simulink model "fft32kpt_ssr32_float"  (R2024a)
settings: Solver=VariableStepAuto  StartTime=0.0  StopTime=sample_period*N*6  RelTol=1e-3
PreLoadFcn:
  | clk_freq = 570e6;
  | SSR=32; % transpose block SSR settings...
  | sample_period = 1/(SSR*clk_freq);
  | N=32768; % fft point size
  | binw=(1/sample_period) / (2*N); % bin width
  | bin_freq = 2*pi*3*binw+pi*binw; % sin, cos freq centered in channel
  | 
  | % for transpose block
  | DATA_WIDTH=32;
  | M=32;
  | N1=N/M;
  | MEM_STYLE=4; % MEM OPTIONS: 4 - ULTRA, 0 - AUTO, 1 - BRAM, 5 - MIXED
InitFcn:
  | clk_freq = 570e6;
  | SSR=32; % transpose block SSR settings...
  | sample_period = 1/(SSR*clk_freq);
  | N=32768; % fft point size
  | binw=(1/sample_period) / (2*N); % bin width
  | bin_freq = 2*pi*3*binw+pi*binw; % sin, cos freq centered in channel
  | 
  | % for transpose block
  | DATA_WIDTH=32;
  | M=32;
  | N1=N/M;
  | MEM_STYLE=4; % MEM OPTIONS: 4 - ULTRA, 0 - AUTO, 1 - BRAM, 5 - MIXED
undefined symbols (not defined in the file or in its folder): None, S, vsva2197, xcvc1902
libraries: hdlBasic x139, aieBasic x95, aieUtilities x32, aieDSP x32, hdlUtilities x32, matrix_library x32, hdlSSR x12, hdlDSPIP x1, simulink x1, dspxfrm3 x1, vmcUtilities x1
(part 4 of 4)

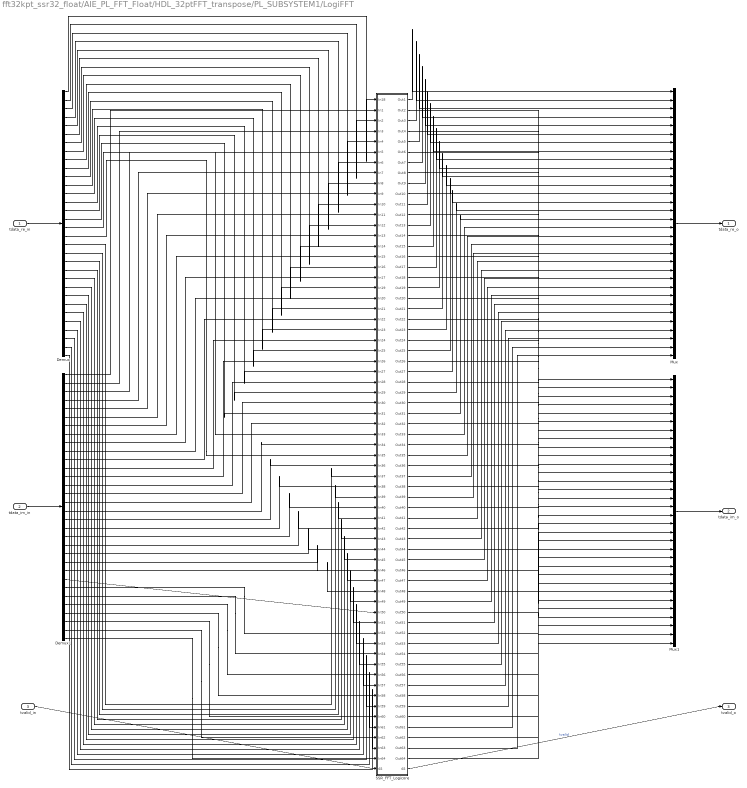
== system fft32kpt_ssr32_float/AIE_PL_FFT_Float/HDL_32ptFFT_transpose/PL_SUBSYSTEM1/LogiFFT ==
  tdata_re_in : Inport
  tdata_im_in : Inport  Port=2
  tvalid_in : Inport  Port=3
  Demux : Demux  Outputs=32
  Demux1 : Demux  Outputs=32
  Mux : Mux  Inputs=32
  Mux1 : Mux  Inputs=32
  SSR_FFT_Logicore : Subsystem
  tdata_re_o : Outport
  tdata_im_o : Outport  Port=2
  tvalid_o : Outport  Port=3
  wires:
  SSR_FFT_Logicore/2(Out2) -> Mux1/1
  SSR_FFT_Logicore/4(Out4) -> Mux1/2
  SSR_FFT_Logicore/6(Out6) -> Mux1/3
  SSR_FFT_Logicore/8(Out8) -> Mux1/4
  SSR_FFT_Logicore/10(Out10) -> Mux1/5
  SSR_FFT_Logicore/12(Out12) -> Mux1/6
  SSR_FFT_Logicore/14(Out14) -> Mux1/7
  SSR_FFT_Logicore/16(Out16) -> Mux1/8
  SSR_FFT_Logicore/18(Out18) -> Mux1/9
  SSR_FFT_Logicore/20(Out20) -> Mux1/10
  SSR_FFT_Logicore/22(Out22) -> Mux1/11
  SSR_FFT_Logicore/24(Out24) -> Mux1/12
  SSR_FFT_Logicore/26(Out26) -> Mux1/13
  SSR_FFT_Logicore/28(Out28) -> Mux1/14
  SSR_FFT_Logicore/30(Out30) -> Mux1/15
  SSR_FFT_Logicore/32(Out32) -> Mux1/16
  SSR_FFT_Logicore/34(Out34) -> Mux1/17
  SSR_FFT_Logicore/36(Out36) -> Mux1/18
  SSR_FFT_Logicore/38(Out38) -> Mux1/19
  SSR_FFT_Logicore/64(Out64) -> Mux1/32
  SSR_FFT_Logicore/40(Out40) -> Mux1/20
  SSR_FFT_Logicore/62(Out62) -> Mux1/31
  SSR_FFT_Logicore/42(Out42) -> Mux1/21
  SSR_FFT_Logicore/60(Out60) -> Mux1/30
  SSR_FFT_Logicore/44(Out44) -> Mux1/22
  SSR_FFT_Logicore/58(Out58) -> Mux1/29
  SSR_FFT_Logicore/46(Out46) -> Mux1/23
  SSR_FFT_Logicore/56(Out56) -> Mux1/28
  SSR_FFT_Logicore/48(Out48) -> Mux1/24
  SSR_FFT_Logicore/54(Out54) -> Mux1/27
  SSR_FFT_Logicore/50(Out50) -> Mux1/25
  SSR_FFT_Logicore/52(Out52) -> Mux1/26
  SSR_FFT_Logicore/63(Out63) -> Mux/32
  SSR_FFT_Logicore/61(Out61) -> Mux/31
  SSR_FFT_Logicore/59(Out59) -> Mux/30
  SSR_FFT_Logicore/57(Out57) -> Mux/29
  SSR_FFT_Logicore/55(Out55) -> Mux/28
  SSR_FFT_Logicore/53(Out53) -> Mux/27
  SSR_FFT_Logicore/51(Out51) -> Mux/26
  SSR_FFT_Logicore/49(Out49) -> Mux/25
  SSR_FFT_Logicore/47(Out47) -> Mux/24
  SSR_FFT_Logicore/45(Out45) -> Mux/23
  SSR_FFT_Logicore/43(Out43) -> Mux/22
  SSR_FFT_Logicore/41(Out41) -> Mux/21
  SSR_FFT_Logicore/39(Out39) -> Mux/20
  SSR_FFT_Logicore/37(Out37) -> Mux/19
  SSR_FFT_Logicore/35(Out35) -> Mux/18
  SSR_FFT_Logicore/33(Out33) -> Mux/17
  SSR_FFT_Logicore/31(Out31) -> Mux/16
  SSR_FFT_Logicore/29(Out29) -> Mux/15
  SSR_FFT_Logicore/27(Out27) -> Mux/14
  SSR_FFT_Logicore/25(Out25) -> Mux/13
  SSR_FFT_Logicore/23(Out23) -> Mux/12
  SSR_FFT_Logicore/21(Out21) -> Mux/11
  SSR_FFT_Logicore/19(Out19) -> Mux/10
  SSR_FFT_Logicore/17(Out17) -> Mux/9
  SSR_FFT_Logicore/15(Out15) -> Mux/8
  SSR_FFT_Logicore/13(Out13) -> Mux/7
  SSR_FFT_Logicore/11(Out11) -> Mux/6
  SSR_FFT_Logicore/9(Out9) -> Mux/5
  SSR_FFT_Logicore/7(Out7) -> Mux/4
  SSR_FFT_Logicore/5(Out5) -> Mux/3
  SSR_FFT_Logicore/3(Out3) -> Mux/2
  SSR_FFT_Logicore/1(Out1) -> Mux/1
  Mux1/1 -> tdata_im_o/1
  Demux1/1 -> SSR_FFT_Logicore/2(In1)
  Demux1/2 -> SSR_FFT_Logicore/4(In3)
  Demux1/3 -> SSR_FFT_Logicore/6(In5)
  Demux1/4 -> SSR_FFT_Logicore/8(In7)
  Demux1/5 -> SSR_FFT_Logicore/10(In9)
  Demux1/6 -> SSR_FFT_Logicore/12(In11)
  Demux1/7 -> SSR_FFT_Logicore/14(In13)
  Demux1/8 -> SSR_FFT_Logicore/16(In15)
  Demux1/9 -> SSR_FFT_Logicore/18(In17)
  Demux1/10 -> SSR_FFT_Logicore/20(In20)
  Demux1/11 -> SSR_FFT_Logicore/22(In22)
  Demux1/12 -> SSR_FFT_Logicore/24(In24)
  Demux1/13 -> SSR_FFT_Logicore/26(In26)
  Demux1/14 -> SSR_FFT_Logicore/28(In28)
  Demux1/15 -> SSR_FFT_Logicore/30(In30)
  Demux1/16 -> SSR_FFT_Logicore/32(In32)
  Demux1/17 -> SSR_FFT_Logicore/34(In34)
  Demux1/32 -> SSR_FFT_Logicore/64(In64)
  Demux1/18 -> SSR_FFT_Logicore/36(In36)
  Demux1/31 -> SSR_FFT_Logicore/62(In62)
  Demux1/19 -> SSR_FFT_Logicore/38(In38)
  Demux1/30 -> SSR_FFT_Logicore/60(In60)
  Demux1/20 -> SSR_FFT_Logicore/40(In40)
  Demux1/29 -> SSR_FFT_Logicore/58(In58)
  Demux1/21 -> SSR_FFT_Logicore/42(In42)
  Demux1/28 -> SSR_FFT_Logicore/56(In56)
  Demux1/22 -> SSR_FFT_Logicore/44(In44)
  Demux1/27 -> SSR_FFT_Logicore/54(In54)
  Demux1/23 -> SSR_FFT_Logicore/46(In46)
  Demux1/26 -> SSR_FFT_Logicore/52(In52)
  Demux1/24 -> SSR_FFT_Logicore/48(In48)
  Demux1/25 -> SSR_FFT_Logicore/50(In50)
  Demux/32 -> SSR_FFT_Logicore/63(In63)
  Demux/31 -> SSR_FFT_Logicore/61(In61)
  Demux/30 -> SSR_FFT_Logicore/59(In59)
  Demux/29 -> SSR_FFT_Logicore/57(In57)
  Demux/28 -> SSR_FFT_Logicore/55(In55)
  Demux/27 -> SSR_FFT_Logicore/53(In53)
  Demux/26 -> SSR_FFT_Logicore/51(In51)
  Demux/25 -> SSR_FFT_Logicore/49(In49)
  Demux/24 -> SSR_FFT_Logicore/47(In47)
  Demux/23 -> SSR_FFT_Logicore/45(In45)
  Demux/22 -> SSR_FFT_Logicore/43(In43)
  Demux/21 -> SSR_FFT_Logicore/41(In41)
  Demux/20 -> SSR_FFT_Logicore/39(In39)
  Demux/19 -> SSR_FFT_Logicore/37(In37)
  Demux/18 -> SSR_FFT_Logicore/35(In35)
  Demux/17 -> SSR_FFT_Logicore/33(In33)
  Demux/16 -> SSR_FFT_Logicore/31(In31)
  Demux/15 -> SSR_FFT_Logicore/29(In29)
  Demux/14 -> SSR_FFT_Logicore/27(In27)
  Demux/13 -> SSR_FFT_Logicore/25(In25)
  Demux/12 -> SSR_FFT_Logicore/23(In23)
  Demux/11 -> SSR_FFT_Logicore/21(In21)
  Demux/10 -> SSR_FFT_Logicore/19(In19)
  Demux/9 -> SSR_FFT_Logicore/17(In16)
  Demux/8 -> SSR_FFT_Logicore/15(In14)
  Demux/7 -> SSR_FFT_Logicore/13(In12)
  Demux/6 -> SSR_FFT_Logicore/11(In10)
  Demux/5 -> SSR_FFT_Logicore/9(In8)
  Demux/4 -> SSR_FFT_Logicore/7(In6)
  Demux/3 -> SSR_FFT_Logicore/5(In4)
  Demux/2 -> SSR_FFT_Logicore/3(In2)
  Demux/1 -> SSR_FFT_Logicore/1(In18)
  tdata_im_in/1 -> Demux1/1
  tvalid_in/1 -> SSR_FFT_Logicore/65(tvalid_in)
  tdata_re_in/1 -> Demux/1
  SSR_FFT_Logicore/65(tvalid_o) -> tvalid_o/1  "tvalid"
  Mux/1 -> tdata_re_o/1

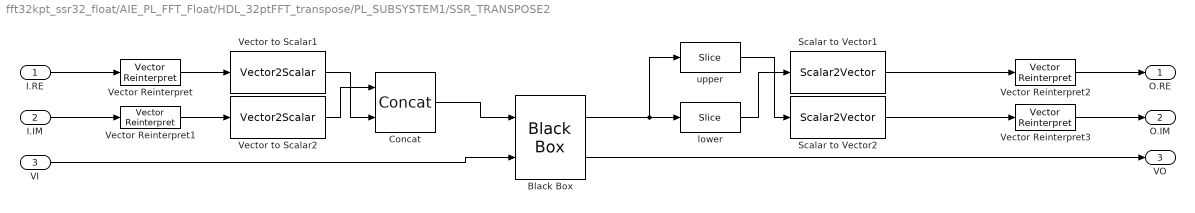
== system fft32kpt_ssr32_float/AIE_PL_FFT_Float/HDL_32ptFFT_transpose/PL_SUBSYSTEM1/SSR_TRANSPOSE2 ==
  "I.RE " : Inport
  "I.IM " : Inport  Port=2
  "VI " : Inport  Port=3
  Black Box : hdlBasic/Black Box  init_code=ssr_transpose_top_config  sim_method=Vivado Simulator  engine_block=../../Questa  verbose=on  XmcBlockStatus=1  maskContainerNames=group1  block_type=blackbox2  block_config=sysgen:black_box_config
  Concat : hdlBasic/Concat  num_inputs=2  XmcBlockStatus=1  maskContainerNames=group1  block_type=concat  block_config=sysgen:Concat_config
  Scalar to Vector1 : hdlSSR/Scalar2Vector  Width=DATA_WIDTH  sg_ssr=SSR  block_type=scalar2vector_ssr  XmcBlockStatus=1  sg_ssr_prev=32  maskContainerNames=group1
  Scalar to Vector2 : hdlSSR/Scalar2Vector  Width=DATA_WIDTH  sg_ssr=SSR  block_type=scalar2vector_ssr  XmcBlockStatus=1  sg_ssr_prev=32  maskContainerNames=group1
  Vector Reinterpret : hdlSSR/Vector Reinterpret  force_arith_type=on  arith_type=Unsigned  force_bin_pt=on  bin_pt=0  sg_ssr=SSR  block_type=reinterpret_ssr  XmcBlockStatus=1  sg_ssr_prev=32  maskContainerNames=group1
  Vector Reinterpret1 : hdlSSR/Vector Reinterpret  force_arith_type=on  arith_type=Unsigned  force_bin_pt=on  bin_pt=0  sg_ssr=SSR  block_type=reinterpret_ssr  XmcBlockStatus=1  sg_ssr_prev=32  maskContainerNames=group1
  Vector Reinterpret2 : hdlSSR/Vector Reinterpret  force_arith_type=on  arith_type=Floating-point  force_bin_pt=on  bin_pt=24  sg_ssr=SSR  block_type=reinterpret_ssr  XmcBlockStatus=1  sg_ssr_prev=32  maskContainerNames=group1
  Vector Reinterpret3 : hdlSSR/Vector Reinterpret  force_arith_type=on  arith_type=Floating-point  force_bin_pt=on  bin_pt=24  sg_ssr=SSR  block_type=reinterpret_ssr  XmcBlockStatus=1  sg_ssr_prev=32  maskContainerNames=group1
  Vector to Scalar1 : hdlSSR/Vector2Scalar  sg_ssr=SSR  block_type=vector2scalar_ssr  XmcBlockStatus=1  sg_ssr_prev=32  maskContainerNames=group1
  Vector to Scalar2 : hdlSSR/Vector2Scalar  sg_ssr=SSR  block_type=vector2scalar_ssr  XmcBlockStatus=1  sg_ssr_prev=32  maskContainerNames=group1
  lower : hdlBasic/Slice  nbits=DATA_WIDTH*SSR  boolean_output=off  mode=Lower Bit Location + Width  bit1=0  base1=MSB of Input  bit0=0  base0=LSB of Input  XmcBlockStatus=1  maskContainerNames=group1  block_type=slice  block_config=sysgen:Slice_config
  upper : hdlBasic/Slice  nbits=DATA_WIDTH*SSR  boolean_output=off  mode=Upper Bit Location + Width  bit1=0  base1=MSB of Input  bit0=0  base0=LSB of Input  XmcBlockStatus=1  maskContainerNames=group1  block_type=slice  block_config=sysgen:Slice_config
  " O.RE" : Outport
  " O.IM" : Outport  Port=2
  " VO" : Outport  Port=3
  wires:
  Vector Reinterpret3/1 -> " O.IM"/1
  Vector Reinterpret2/1 -> " O.RE"/1
  Vector Reinterpret/1 -> Vector to Scalar1/1
  "VI "/1 -> Black Box/2
  Vector to Scalar1/1 -> Concat/2
  lower/1 -> Scalar to Vector1/1
  upper/1 -> Scalar to Vector2/1
  Black Box/1 -> lower/1, upper/1
  Vector to Scalar2/1 -> Concat/1
  Concat/1 -> Black Box/1
  Vector Reinterpret1/1 -> Vector to Scalar2/1
  Black Box/2 -> " VO"/1
  Scalar to Vector1/1 -> Vector Reinterpret2/1
  Scalar to Vector2/1 -> Vector Reinterpret3/1
  "I.RE "/1 -> Vector Reinterpret/1
  "I.IM "/1 -> Vector Reinterpret1/1

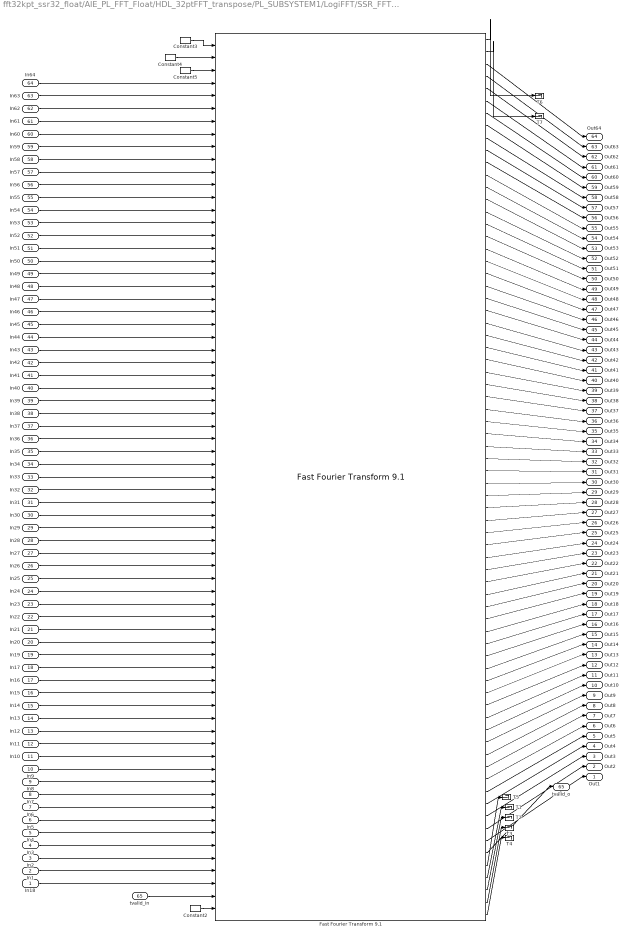
== system fft32kpt_ssr32_float/AIE_PL_FFT_Float/HDL_32ptFFT_transpose/PL_SUBSYSTEM1/LogiFFT/SSR_FFT_Logicore ==
  In18 : Inport
  In1 : Inport  Port=2
  In2 : Inport  Port=3
  In3 : Inport  Port=4
  In4 : Inport  Port=5
  In5 : Inport  Port=6
  In6 : Inport  Port=7
  In7 : Inport  Port=8
  In8 : Inport  Port=9
  In9 : Inport  Port=10
  In10 : Inport  Port=11
  In11 : Inport  Port=12
  In12 : Inport  Port=13
  In13 : Inport  Port=14
  In14 : Inport  Port=15
  In15 : Inport  Port=16
  In16 : Inport  Port=17
  In17 : Inport  Port=18
  In19 : Inport  Port=19
  In20 : Inport  Port=20
  In21 : Inport  Port=21
  In22 : Inport  Port=22
  In23 : Inport  Port=23
  In24 : Inport  Port=24
  In25 : Inport  Port=25
  In26 : Inport  Port=26
  In27 : Inport  Port=27
  In28 : Inport  Port=28
  In29 : Inport  Port=29
  In30 : Inport  Port=30
  In31 : Inport  Port=31
  In32 : Inport  Port=32
  In33 : Inport  Port=33
  In34 : Inport  Port=34
  In35 : Inport  Port=35
  In36 : Inport  Port=36
  In37 : Inport  Port=37
  In38 : Inport  Port=38
  In39 : Inport  Port=39
  In40 : Inport  Port=40
  In41 : Inport  Port=41
  In42 : Inport  Port=42
  In43 : Inport  Port=43
  In44 : Inport  Port=44
  In45 : Inport  Port=45
  In46 : Inport  Port=46
  In47 : Inport  Port=47
  In48 : Inport  Port=48
  In49 : Inport  Port=49
  In50 : Inport  Port=50
  In51 : Inport  Port=51
  In52 : Inport  Port=52
  In53 : Inport  Port=53
  In54 : Inport  Port=54
  In55 : Inport  Port=55
  In56 : Inport  Port=56
  In57 : Inport  Port=57
  In58 : Inport  Port=58
  In59 : Inport  Port=59
  In60 : Inport  Port=60
  In61 : Inport  Port=61
  In62 : Inport  Port=62
  In63 : Inport  Port=63
  In64 : Inport  Port=64
  tvalid_in : Inport  Port=65
  Constant2 : hdlBasic/Constant  const=0  gui_display_data_type=Boolean  arith_type=Boolean  n_bits=16  bin_pt=14  preci_type=Single  exp_width=8  frac_width=24  explicit_period=off  period=1  XmcBlockStatus=1  maskContainerNames=tabcontainer1  block_type=constant  block_config=sysgen:Constant_config
  Constant3 : hdlBasic/Constant  const=0  gui_display_data_type=Fixed-point  arith_type=Unsigned  n_bits=6  bin_pt=0  preci_type=Single  exp_width=8  frac_width=24  explicit_period=off  period=1  XmcBlockStatus=1  maskContainerNames=tabcontainer1  block_type=constant  block_config=sysgen:Constant_config
  Constant4 : hdlBasic/Constant  const=1.0  gui_display_data_type=Fixed-point  arith_type=Unsigned  n_bits=1  bin_pt=0  preci_type=Single  exp_width=8  frac_width=24  explicit_period=off  period=1  XmcBlockStatus=1  maskContainerNames=tabcontainer1  block_type=constant  block_config=sysgen:Constant_config
  Constant5 : hdlBasic/Constant  const=0  gui_display_data_type=Boolean  arith_type=Boolean  n_bits=16  bin_pt=14  preci_type=Single  exp_width=8  frac_width=24  explicit_period=off  period=1  XmcBlockStatus=1  maskContainerNames=tabcontainer1  block_type=constant  block_config=sysgen:Constant_config
  Fast Fourier Transform 9.1 : hdlDSPIP/Fast Fourier Transform 9.1   transform_length=32  target_clock_frequency=clk_freq/1e6  target_data_throughput=clk_freq/1e6  implementation_options=automatically_select  run_time_configurable_transform_length=off  enable_ssr=on  super_sample_rates=32  data_format=native_floating_point  phase_factor_width=18  scaling_options=scaled  rounding_modes=truncation  aclken=off  aresetn=off  output_ordering=bit_reversed_order  cyclic_prefix_insertion=off  throttle_scheme=realtime  xk_index=off  ovflo=off  trim_axipin_name=on  memory_options_data=block_ram  memory_options_phase_factors=block_ram  number_of_stages_using_block_ram_for_data_and_phase_factors=0  memory_options_reorder=block_ram  memory_options_hybrid=off  complex_mult_type=use_mults_resources  butterfly_type=use_luts  simulation_type=hybrid  simulation_model=sysgen:xfftv9_cmodel  data_path_portlist={ 's_axis_data_tdata', 'm_axis_data_tdata', 'm_axis_status_tdata', 'event_fft_overflow' }  channels=1  input_ordering=natural_order  input_width=16  ip_name=Fast Fourier Transform  ip_version=9.1  dsptool_ready=true  ipcore_usecache=true  ipcore_useipmodelcache=true  wrapper_available=true  port_translation_map={ 'aclken' => 'en', 'aresetn' => 'rst'}  XmcBlockStatus=1  maskContainerNames=tabcontainer1  block_type=xfft_v9_1  block_config=sysgen:rodinimport_config
  T{1..7} (7 alike) : Terminator
  Out1 : Outport
  Out2 : Outport  Port=2
  Out3 : Outport  Port=3
  Out4 : Outport  Port=4
  Out5 : Outport  Port=5
  Out6 : Outport  Port=6
  Out7 : Outport  Port=7
  Out8 : Outport  Port=8
  Out9 : Outport  Port=9
  Out10 : Outport  Port=10
  Out11 : Outport  Port=11
  Out12 : Outport  Port=12
  Out13 : Outport  Port=13
  Out14 : Outport  Port=14
  Out15 : Outport  Port=15
  Out16 : Outport  Port=16
  Out17 : Outport  Port=17
  Out18 : Outport  Port=18
  Out19 : Outport  Port=19
  Out20 : Outport  Port=20
  Out21 : Outport  Port=21
  Out22 : Outport  Port=22
  Out23 : Outport  Port=23
  Out24 : Outport  Port=24
  Out25 : Outport  Port=25
  Out26 : Outport  Port=26
  Out27 : Outport  Port=27
  Out28 : Outport  Port=28
  Out29 : Outport  Port=29
  Out30 : Outport  Port=30
  Out31 : Outport  Port=31
  Out32 : Outport  Port=32
  Out33 : Outport  Port=33
  Out34 : Outport  Port=34
  Out35 : Outport  Port=35
  Out36 : Outport  Port=36
  Out37 : Outport  Port=37
  Out38 : Outport  Port=38
  Out39 : Outport  Port=39
  Out40 : Outport  Port=40
  Out41 : Outport  Port=41
  Out42 : Outport  Port=42
  Out43 : Outport  Port=43
  Out44 : Outport  Port=44
  Out45 : Outport  Port=45
  Out46 : Outport  Port=46
  Out47 : Outport  Port=47
  Out48 : Outport  Port=48
  Out49 : Outport  Port=49
  Out50 : Outport  Port=50
  Out51 : Outport  Port=51
  Out52 : Outport  Port=52
  Out53 : Outport  Port=53
  Out54 : Outport  Port=54
  Out55 : Outport  Port=55
  Out56 : Outport  Port=56
  Out57 : Outport  Port=57
  Out58 : Outport  Port=58
  Out59 : Outport  Port=59
  Out60 : Outport  Port=60
  Out61 : Outport  Port=61
  Out62 : Outport  Port=62
  Out63 : Outport  Port=63
  Out64 : Outport  Port=64
  tvalid_o : Outport  Port=65
  wires:
  Fast Fourier Transform 9.1/66 -> Out1/1
  Fast Fourier Transform 9.1/65 -> Out2/1
  Fast Fourier Transform 9.1/64 -> Out3/1
  Fast Fourier Transform 9.1/63 -> Out4/1
  Fast Fourier Transform 9.1/62 -> Out5/1
  Fast Fourier Transform 9.1/61 -> Out6/1
  Fast Fourier Transform 9.1/60 -> Out7/1
  Fast Fourier Transform 9.1/59 -> Out8/1
  Fast Fourier Transform 9.1/58 -> Out9/1
  Fast Fourier Transform 9.1/57 -> Out10/1
  Fast Fourier Transform 9.1/56 -> Out11/1
  Fast Fourier Transform 9.1/55 -> Out12/1
  Fast Fourier Transform 9.1/54 -> Out13/1
  Fast Fourier Transform 9.1/53 -> Out14/1
  Fast Fourier Transform 9.1/52 -> Out15/1
  Fast Fourier Transform 9.1/51 -> Out16/1
  Fast Fourier Transform 9.1/50 -> Out17/1
  Fast Fourier Transform 9.1/49 -> Out18/1
  Fast Fourier Transform 9.1/48 -> Out19/1
  Fast Fourier Transform 9.1/47 -> Out20/1
  Fast Fourier Transform 9.1/46 -> Out21/1
  Fast Fourier Transform 9.1/45 -> Out22/1
  Fast Fourier Transform 9.1/44 -> Out23/1
  Fast Fourier Transform 9.1/43 -> Out24/1
  Fast Fourier Transform 9.1/42 -> Out25/1
  Fast Fourier Transform 9.1/41 -> Out26/1
  Fast Fourier Transform 9.1/40 -> Out27/1
  Fast Fourier Transform 9.1/39 -> Out28/1
  Fast Fourier Transform 9.1/38 -> Out29/1
  Fast Fourier Transform 9.1/37 -> Out30/1
  Fast Fourier Transform 9.1/36 -> Out31/1
  Fast Fourier Transform 9.1/35 -> Out32/1
  Fast Fourier Transform 9.1/34 -> Out33/1
  Fast Fourier Transform 9.1/33 -> Out34/1
  Fast Fourier Transform 9.1/32 -> Out35/1
  Fast Fourier Transform 9.1/31 -> Out36/1
  Fast Fourier Transform 9.1/30 -> Out37/1
  Fast Fourier Transform 9.1/29 -> Out38/1
  Fast Fourier Transform 9.1/28 -> Out39/1
  Fast Fourier Transform 9.1/27 -> Out40/1
  Fast Fourier Transform 9.1/26 -> Out41/1
  Fast Fourier Transform 9.1/25 -> Out42/1
  Fast Fourier Transform 9.1/24 -> Out43/1
  Fast Fourier Transform 9.1/23 -> Out44/1
  Fast Fourier Transform 9.1/22 -> Out45/1
  Fast Fourier Transform 9.1/21 -> Out46/1
  Fast Fourier Transform 9.1/20 -> Out47/1
  Fast Fourier Transform 9.1/19 -> Out48/1
  Fast Fourier Transform 9.1/18 -> Out49/1
  Fast Fourier Transform 9.1/17 -> Out50/1
  Fast Fourier Transform 9.1/16 -> Out51/1
  Fast Fourier Transform 9.1/15 -> Out52/1
  Fast Fourier Transform 9.1/14 -> Out53/1
  Fast Fourier Transform 9.1/13 -> Out54/1
  Fast Fourier Transform 9.1/12 -> Out55/1
  Fast Fourier Transform 9.1/11 -> Out56/1
  Fast Fourier Transform 9.1/10 -> Out57/1
  Fast Fourier Transform 9.1/9 -> Out58/1
  Fast Fourier Transform 9.1/8 -> Out59/1
  Fast Fourier Transform 9.1/7 -> Out60/1
  Fast Fourier Transform 9.1/6 -> Out61/1
  Fast Fourier Transform 9.1/5 -> Out62/1
  Fast Fourier Transform 9.1/4 -> Out63/1
  Fast Fourier Transform 9.1/3 -> Out64/1
  tvalid_in/1 -> Fast Fourier Transform 9.1/68
  In18/1 -> Fast Fourier Transform 9.1/67
  In1/1 -> Fast Fourier Transform 9.1/66
  In2/1 -> Fast Fourier Transform 9.1/65
  In3/1 -> Fast Fourier Transform 9.1/64
  In4/1 -> Fast Fourier Transform 9.1/63
  In5/1 -> Fast Fourier Transform 9.1/62
  In6/1 -> Fast Fourier Transform 9.1/61
  In7/1 -> Fast Fourier Transform 9.1/60
  In8/1 -> Fast Fourier Transform 9.1/59
  In9/1 -> Fast Fourier Transform 9.1/58
  In10/1 -> Fast Fourier Transform 9.1/57
  In11/1 -> Fast Fourier Transform 9.1/56
  In12/1 -> Fast Fourier Transform 9.1/55
  In13/1 -> Fast Fourier Transform 9.1/54
  In14/1 -> Fast Fourier Transform 9.1/53
  In15/1 -> Fast Fourier Transform 9.1/52
  In16/1 -> Fast Fourier Transform 9.1/51
  In17/1 -> Fast Fourier Transform 9.1/50
  In19/1 -> Fast Fourier Transform 9.1/49
  In20/1 -> Fast Fourier Transform 9.1/48
  In21/1 -> Fast Fourier Transform 9.1/47
  In22/1 -> Fast Fourier Transform 9.1/46
  In23/1 -> Fast Fourier Transform 9.1/45
  In24/1 -> Fast Fourier Transform 9.1/44
  In25/1 -> Fast Fourier Transform 9.1/43
  In26/1 -> Fast Fourier Transform 9.1/42
  In27/1 -> Fast Fourier Transform 9.1/41
  In28/1 -> Fast Fourier Transform 9.1/40
  In29/1 -> Fast Fourier Transform 9.1/39
  In30/1 -> Fast Fourier Transform 9.1/38
  In31/1 -> Fast Fourier Transform 9.1/37
  In32/1 -> Fast Fourier Transform 9.1/36
  In33/1 -> Fast Fourier Transform 9.1/35
  In34/1 -> Fast Fourier Transform 9.1/34
  In35/1 -> Fast Fourier Transform 9.1/33
  In36/1 -> Fast Fourier Transform 9.1/32
  In37/1 -> Fast Fourier Transform 9.1/31
  In38/1 -> Fast Fourier Transform 9.1/30
  In39/1 -> Fast Fourier Transform 9.1/29
  In40/1 -> Fast Fourier Transform 9.1/28
  In41/1 -> Fast Fourier Transform 9.1/27
  In42/1 -> Fast Fourier Transform 9.1/26
  In43/1 -> Fast Fourier Transform 9.1/25
  In44/1 -> Fast Fourier Transform 9.1/24
  In45/1 -> Fast Fourier Transform 9.1/23
  In46/1 -> Fast Fourier Transform 9.1/22
  In47/1 -> Fast Fourier Transform 9.1/21
  In48/1 -> Fast Fourier Transform 9.1/20
  In49/1 -> Fast Fourier Transform 9.1/19
  In50/1 -> Fast Fourier Transform 9.1/18
  In51/1 -> Fast Fourier Transform 9.1/17
  In52/1 -> Fast Fourier Transform 9.1/16
  In53/1 -> Fast Fourier Transform 9.1/15
  In54/1 -> Fast Fourier Transform 9.1/14
  In55/1 -> Fast Fourier Transform 9.1/13
  In56/1 -> Fast Fourier Transform 9.1/12
  In57/1 -> Fast Fourier Transform 9.1/11
  In58/1 -> Fast Fourier Transform 9.1/10
  In59/1 -> Fast Fourier Transform 9.1/9
  In60/1 -> Fast Fourier Transform 9.1/8
  In61/1 -> Fast Fourier Transform 9.1/7
  In62/1 -> Fast Fourier Transform 9.1/6
  In63/1 -> Fast Fourier Transform 9.1/5
  In64/1 -> Fast Fourier Transform 9.1/4
  Fast Fourier Transform 9.1/1 -> T6/1
  Fast Fourier Transform 9.1/2 -> T7/1
  Fast Fourier Transform 9.1/68 -> T5/1
  Fast Fourier Transform 9.1/69 -> T1/1
  Fast Fourier Transform 9.1/70 -> T2/1
  Fast Fourier Transform 9.1/71 -> T3/1
  Fast Fourier Transform 9.1/72 -> T4/1
  Constant2/1 -> Fast Fourier Transform 9.1/69
  Constant5/1 -> Fast Fourier Transform 9.1/3
  Fast Fourier Transform 9.1/67 -> tvalid_o/1
  Constant4/1 -> Fast Fourier Transform 9.1/2
  Constant3/1 -> Fast Fourier Transform 9.1/1
